simulink model "continental_test"  (R2014a)
settings: Solver=ode45  StartTime=0.0  StopTime=50  RelTol=1e-4
InitFcn:
  | run('head_test.m')
undefined symbols (not defined in the file or in its folder): car
settings Model: Creator=WXY  LastModifiedBy=WXY

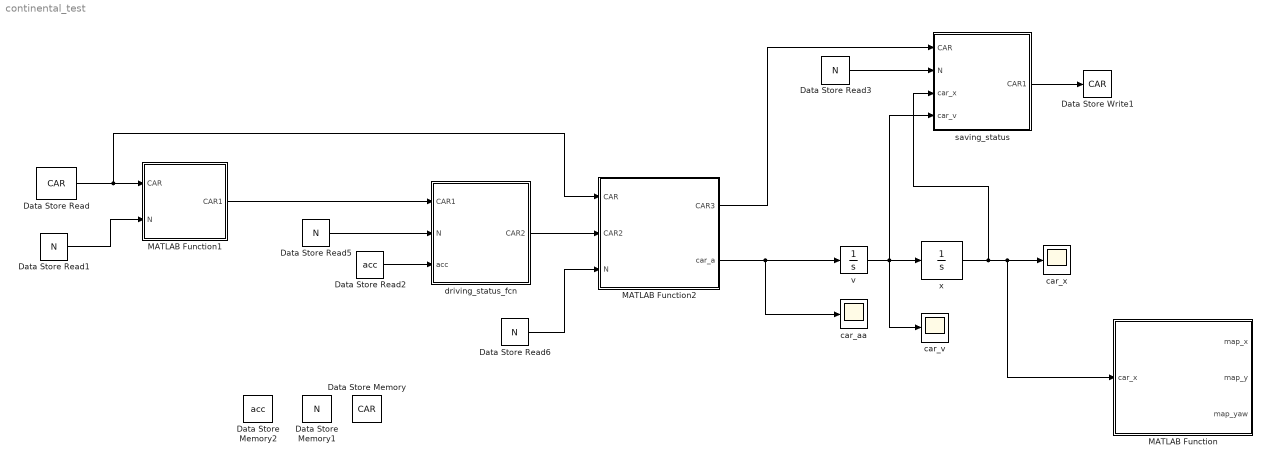
== system continental_test ==
  Data Store Memory : DataStoreMemory  DataStoreName=CAR  ReadBeforeWriteMsg=warning  WriteAfterWriteMsg=warning  WriteAfterReadMsg=warning  InitialValue=car  VectorParams1D=off
  Data Store Memory1 : DataStoreMemory  DataStoreName=N  ReadBeforeWriteMsg=warning  WriteAfterWriteMsg=warning  WriteAfterReadMsg=warning  InitialValue=N
  Data Store Memory2 : DataStoreMemory  DataStoreName=acc  ReadBeforeWriteMsg=warning  WriteAfterWriteMsg=warning  WriteAfterReadMsg=warning  InitialValue=acc
  Data Store Read : DataStoreRead  DataStoreName=CAR
  Data Store Read{1,3,5..6} (4 alike) : DataStoreRead  DataStoreName=N
  Data Store Read2 : DataStoreRead  DataStoreName=acc
  Data Store Write1 : DataStoreWrite  DataStoreName=CAR
  MATLAB Function : MATLAB Function  TreatAsAtomicUnit=on
  MATLAB Function1 : MATLAB Function  TreatAsAtomicUnit=on
  MATLAB Function2 : MATLAB Function  TreatAsAtomicUnit=on
  car_aa : Scope
      settings: YMin=-22  YMax=1  SaveName=ScopeData4
  car_v : Scope
      settings: TimeRange=50  YMin=-17.5  YMax=17.5  SaveName=ScopeData2
  car_x : Scope
      settings: YMin=0  YMax=325
  driving_status_fcn : MATLAB Function  TreatAsAtomicUnit=on
  saving_status : MATLAB Function  TreatAsAtomicUnit=on
  v : Integrator  InitialCondition=car(:,2)'
  x : Integrator  InitialCondition=car(:,1)'
  wires:
  v/1 -> saving_status/4(car_v), car_v/1, x/1
  x/1 -> MATLAB Function/1(car_x), car_x/1, saving_status/3(car_x)
  Data Store Read2/1 -> driving_status_fcn/3(acc)
  Data Store Read3/1 -> saving_status/2(N)
  saving_status/1(CAR1) -> Data Store Write1/1
  Data Store Read/1 -> MATLAB Function2/1(CAR), MATLAB Function1/1(CAR)
  Data Store Read1/1 -> MATLAB Function1/2(N)
  MATLAB Function1/1(CAR1) -> driving_status_fcn/1(CAR1)
  Data Store Read5/1 -> driving_status_fcn/2(N)
  driving_status_fcn/1(CAR2) -> MATLAB Function2/2(CAR2)
  Data Store Read6/1 -> MATLAB Function2/3(N)
  MATLAB Function2/1(CAR3) -> saving_status/1(CAR)
  MATLAB Function2/2(car_a) -> car_aa/1, v/1

== matlab function continental_test/saving_status ==
  data: CAR input; CAR1 output; N input; car_x input; car_v input
function CAR1  = fcn(CAR,N,car_x,car_v)
x=1;v=2;
for i=1:N
    CAR(:,x)=car_x';
    CAR(:,v)=car_v';
end


 CAR1=CAR;

end

== matlab function continental_test/driving_status_fcn ==
  data: CAR1 input; CAR2 output; N input; acc input
function CAR2  = fcn(CAR1,N,acc)
x=1;v=2;a=3;v_suggest=4;
%找CAR1中有多少有效信息
count=0;
for i=1:3
   if CAR1(i,8)==1 || CAR1(i,8)==0
    count=count+1;
   end
end
N=count;
%车辆之间互相判断
if N==1
        if  CAR1(1,v)<CAR1(1,v_suggest)
            CAR1(1,a)=acc;
        elseif CAR1(1,v)==CAR1(1,v_suggest)
            CAR1(1,a)=0;
        else
            CAR1(1,a)=-acc;
        end  
else
    for i=1:N-1
        if CAR1(i,v)<=CAR1(i+1,v_suggest)
            distance=(CAR1(i,x)-CAR1(i+1,x));
            if distance>50
                if  CAR1(i+1,v)<CAR1(i+1,v_suggest)
                    CAR1(i+1,a)=acc;
                elseif CAR1(i+1,v)==CAR1(i+1,v_suggest)
                    CAR1(i+1,a)=0;
                else
                    CAR1(i+1,a)=-acc;
                end
            else
                CAR1(i+1,a)=0;
                safty_distance=((CAR1(i+1,v))^2-(CAR1(i,v))^2)/(2*acc)+3;  %安全距离
                if safty_distance>(CAR1(i,x)-CAR1(i+1,x))  %后面车辆有撞击可能性，但直到小于安全距离才刹车
                    CAR1(i+1,a)=-acc;
                    if CAR1(i,v)>=CAR1(i+1,v)
                        CAR1(i+1,a)=0;
                    end
                end
            end
        else
            if  CAR1(i+1,v)<CAR1(i+1,v_suggest)
                CAR1(i+1,a)=acc;
            elseif CAR1(i+1,v)==CAR1(i+1,v_suggest)
                CAR1(i+1,a)=0;
            else
                CAR1(i+1,a)=-acc;
            end
        end
    end
end

CAR2=CAR1;
end

== matlab function continental_test/MATLAB Function ==
  data: car_x input; map_x output; map_y output; map_yaw output
function [map_x,map_y,map_yaw] = fcn(car_x)
map_x=zeros(3,1);map_y=zeros(3,1);map_yaw=zeros(3,1);
Light_location=[0,132,224,356]; %红绿灯位置
car_num=size(car_x); %有几辆车
car_road_position=zeros(10,1);



for i=1:car_num(1)
   count=1;
   while(~( car_x(i)>=Light_location(count) && car_x(i)<Light_location(count+1) )) 
       %如果车辆不在这段路的节点之间，则进入该循环
       count=count+1;
   end
   car_road_position(i)=count; %记录第i辆车在哪一段路上
end

%得到每辆车在哪一段路上过后，开始重新计算坐标
for i=1:car_num(1)
   switch car_road_position(i)
       case 1
         map_x(i)=car_x(i);
         map_y(i)=0;
         map_yaw(i)=0;
       case 2
           map_x(i)=Light_location(2);
         map_y(i)=car_x(i)-Light_location(2);
         map_yaw(i)=-90;
       case 3
         map_x(i)=Light_location(3);
         map_y(i)=car_x(i)-Light_location(3);
         map_yaw(i)=0;
       otherwise
           map_x(i)=car_x(i);
           map_y(i)=0;
           map_yaw(i)=0;
   end
    
end



end

== matlab function continental_test/MATLAB Function1 ==
  data: CAR input; CAR1 output; N input
function CAR1 = fcn(CAR,N)
CAR1=ones(3,8)-100;
%提取主车和客车到CAR1
for i=1:N
   if CAR(i,8)==1 ||CAR(i,8)==0
    CAR1(i,:)=CAR(i,:);
   end
end   

%对CAR1按照x进行降序排列
CAR1=sortrows(CAR1,-1);
end

== matlab function continental_test/MATLAB Function2 ==
  data: CAR input; CAR2 input; CAR3 output; N input; car_a output
function [CAR3,car_a] = fcn(CAR,CAR2,N)

for i=1:N
   for j=1:N
      if CAR2(i,7)==CAR(j,7)
          CAR(j,:)=CAR2(i,:);
      end
   end
end
CAR3=CAR;
car_a=CAR3(:,3)';
end
